simulink model "testing_C_functions_doubles3"  (R2020b)
settings: Solver=VariableStepAuto  StartTime=0.0  StopTime=2  FixedStep=Ts
undefined symbols (not defined in the file or in its folder): A_frq_step, A_phase_step, DiscIntNeverNeededParam, f_rad, k_phi, ki, kp, N, t_frq_step, t_phase_step, Ts, V_g, var_noise
libraries: simulink x9, bach_library x3, dspsrcs4 x2
settings Model: Creator=Kasper Laustsen  LastModifiedBy=Kasper Laustsen
settings SFSimCC: SimCustomHeaderCode=|
  | #include "PLL_doubled.h"
  | #include "MAF_doubled.h"
settings SFSimCC: SimUserSources=|
  | PLL_doubled.c
  | MAF_doubled.c

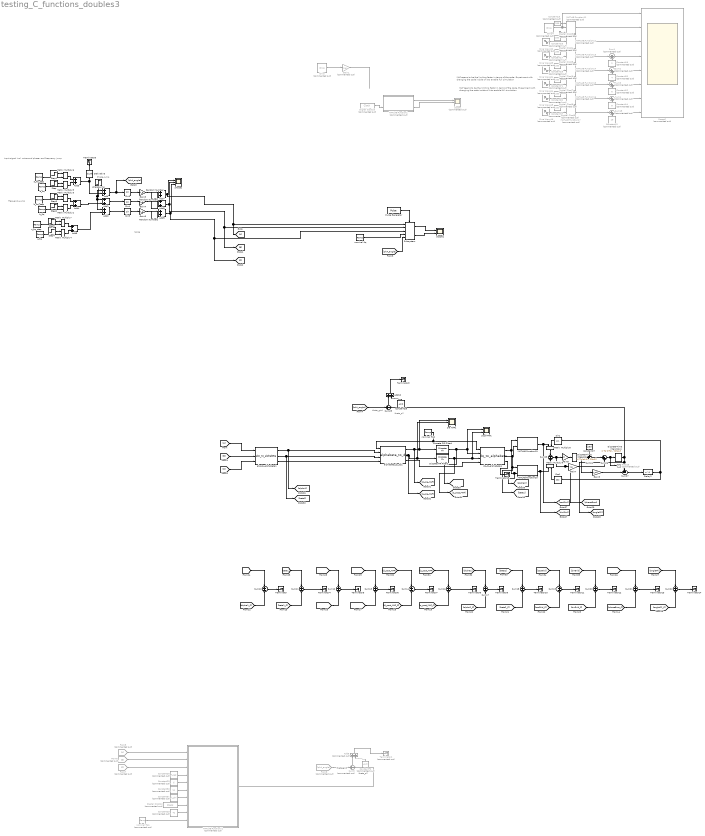
== system testing_C_functions_doubles3 ==
  note: MAF seems to be the limiting factor in terms of the code.
      | Experiment with changing the code inside of it to enable full simulation
  note: Noise
  note: Phase-jump
  note: Input signal incl. noise and phase- and frequency jump
  note: Frequency-jump
  note: MAF seems to be the limiting factor in terms of the code.
      | Experiment with changing the code inside of it to enable full simulation
  note: theta_pll
  note: theta_grid
  note: theta_pll
  note: theta_grid
  Add{,1..5,7..10} (10 alike) : Sum
  Add6 : Sum  Commented=on
  Chirp : dspsrcs4/Chirp  Commented=on  sweep=Linear  mode=Unidirectional  f0=0  f1=150  t1=3  Tsweep=3  phase=0  Ts=Ts  spf=1  datatype=Double  OutputFrames=off
  Chirp4 : dspsrcs4/Chirp  Commented=on  sweep=Linear  mode=Bidirectional  f0=0  f1=100  t1=2  Tsweep=2  phase=0  Ts=Ts  spf=1  datatype=Single  OutputFrames=off
  Constant12 : Constant  Commented=on  Value=6
  Constant13 : Constant  Commented=on  Value=10
  Constant14 : Constant  Commented=on  Value=8
  Constant{15..18,21..23} (7 alike) : Constant  Commented=on  Value=200
  Constant19 : Constant  Commented=on  Value=2
  Constant20 : Constant  Commented=on  Value=4
  Constant25 : Constant  Commented=on  Value=Ts
  Constant26 : Constant  Commented=on  Value=f_rad
  Constant27 : Constant  Value=f_rad
  Constant28 : Constant  Value=-pi/2
  Constant29 : Constant  Commented=on  Value=ki
  Constant30 : Constant  Commented=on  Value=kp
  Constant31 : Constant  Commented=on  Value=k_phi
  Constant32 : Constant  Commented=on  Value=-pi/2
  Cos1 : Trigonometry  Operator=cos
  Delay2 : Delay  DelayLength=1
  Derivative : Derivative
  Digital Clock{3..10,12} (9 alike) : DigitalClock  Commented=on  SampleTime=Ts
  Discrete FIR Filter2 : DiscreteFir  Coefficients=[ones(1,round(N)).*1/N]  SampleTime=Ts
  Discrete FIR Filter4 : DiscreteFir  Coefficients=[ones(1,round(N)).*1/N]  SampleTime=Ts
  Discrete-Time Integrator3 : DiscreteIntegrator  IntegratorMethod=Integration: Trapezoidal  SampleTime=-1  ICPrevOutput=DiscIntNeverNeededParam  ICPrevScaledInput=DiscIntNeverNeededParam
  Discrete-Time Integrator4 : DiscreteIntegrator  IntegratorMethod=Integration: Trapezoidal  SampleTime=-1  ICPrevOutput=DiscIntNeverNeededParam  ICPrevScaledInput=DiscIntNeverNeededParam
  From5 : From  Commented=on
  From6 : From  Commented=on  GotoTag=B
  From7 : From  Commented=on  GotoTag=C
  From8 : From  Commented=on  GotoTag=phA_angle
  Gain1 : Gain  Commented=on  Gain=V_g
  Gain3 : Gain  Gain=V_g
  Gain4 : Gain  Gain=V_g
  Gain5 : Gain  Gain=V_g
  Gain7 : Gain  Gain=kp
  Gain8 : Gain  Gain=ki
  Gain9 : Gain  Gain=k_phi
  Goto25 : Goto  Commented=on
  MATLAB Function1 : MATLAB Function  Commented=on  TreatAsAtomicUnit=on
  MATLAB Function11 : MATLAB Function  Commented=on  TreatAsAtomicUnit=on
  MATLAB Function12 : MATLAB Function  Commented=on  TreatAsAtomicUnit=on
  MATLAB Function13 : MATLAB Function  Commented=on  TreatAsAtomicUnit=on
  MATLAB Function14 : MATLAB Function  Commented=on  TreatAsAtomicUnit=on
  MATLAB Function15 : MATLAB Function  Commented=on  TreatAsAtomicUnit=on
  MATLAB Function16 : MATLAB Function  Commented=on  TreatAsAtomicUnit=on
  MATLAB Function17 : MATLAB Function  Commented=on  TreatAsAtomicUnit=on
  MATLAB Function19 : MATLAB Function  TreatAsAtomicUnit=on
  MATLAB Function20 : MATLAB Function  TreatAsAtomicUnit=on
  MATLAB Function21 : MATLAB Function  Commented=on  TreatAsAtomicUnit=on
  Matrix Multiply{2..9} (8 alike) : Product
  Pulse Generator : DiscretePulseGenerator  PulseType=Time based  Period=Ts  PulseWidth=50
  Random Number : RandomNumber  Variance=var_noise  SampleTime=Ts
  Random Number1 : RandomNumber  Variance=var_noise  Seed=1  SampleTime=Ts
  Random Number2 : RandomNumber  Variance=var_noise  Seed=2  SampleTime=Ts
  Scope : Scope  Commented=on  NumInputPorts=3
  Scope1 : Scope  NumInputPorts=2
  Scope2 : Scope  Commented=on  NumInputPorts=8
  Sin{1,3..5} (4 alike) : Trigonometry
  Sine Wave14 : Sin  Commented=on  Frequency=f_rad*2.6  Phase=pi/2  SampleTime=Ts
  Sine Wave15 : Sin  Commented=on  Frequency=f_rad*2.8  Phase=pi/2  SampleTime=Ts
  Sine Wave16 : Sin  Commented=on  Frequency=f_rad*3  Phase=pi/2  SampleTime=Ts
  Sine Wave22 : Sin  Commented=on  Frequency=f_rad*2  Phase=pi/2  SampleTime=Ts
  Sine Wave23 : Sin  Commented=on  Frequency=f_rad*2.2  Phase=pi/2  SampleTime=Ts
  Sine Wave24 : Sin  Commented=on  Frequency=f_rad*2.4  Phase=pi/2  SampleTime=Ts
  Step : Step  Time=t_frq_step  Before=1  After=0  SampleTime=0
  Step1 : Step  Time=t_frq_step  SampleTime=0
  Step2 : Step  Time=t_frq_step  Before=1  After=0  SampleTime=0
  Step3 : Step  Time=t_frq_step  SampleTime=0
  Step4 : Step  Time=t_frq_step  Before=1  After=0  SampleTime=0
  Step5 : Step  Time=t_frq_step  SampleTime=0
  Subsystem : Subsystem
  Sum{1..4,15} (5 alike) : Sum  Commented=on  Inputs=|++
  Sum{10..14,16..22,25} (13 alike) : Sum  Inputs=+|-
  Sum23 : Sum  Inputs=-|+
  Sum24 : Sum  Inputs=++|
  Sum26 : Sum  Inputs=|++
  Sum27 : Sum  Inputs=+-|
  Sum5 : Sum  Commented=on  Inputs=+|-
  Terminator{,2..15} (15 alike) : Terminator
  Terminator1 : Terminator  Commented=on
  a_frq : simulink/Sources/Ramp  slope=f_rad  start=0  InitialOutput=0
  a_frq_step : simulink/Sources/Ramp  slope=f_rad*A_frq_step  start=t_frq_step  InitialOutput=t_frq_step*f_rad
  abc_to_alphabeta1 : bach_library/abc_to_alphabeta  SystemSampleTime=-1  VariantActivationTime=update diagram  Latency=0  AutoFrameSizeCalculation=off
  alphabeta_to_dq1 : bach_library/alphabeta_to_dq  SystemSampleTime=-1  VariantActivationTime=update diagram  Latency=0  AutoFrameSizeCalculation=off
  b_frq : simulink/Sources/Ramp  slope=f_rad  start=0  InitialOutput=-pi*2/3
  b_frq_step : simulink/Sources/Ramp  slope=f_rad*A_frq_step  start=t_frq_step  InitialOutput=t_frq_step*f_rad-pi*2/3
  c_frq : simulink/Sources/Ramp  slope=f_rad  start=0  InitialOutput=pi*2/3
  c_frq_step : simulink/Sources/Ramp  slope=f_rad*A_frq_step  start=t_frq_step  InitialOutput=t_frq_step*f_rad+pi*2/3
  dq_to_alphabeta1 : bach_library/dq_to_alphabeta  SystemSampleTime=-1  VariantActivationTime=update diagram  Latency=0  AutoFrameSizeCalculation=off
  nominal frq : simulink/Sources/Ramp  slope=f_rad  start=0  InitialOutput=0
  nominal frq1 : simulink/Sources/Ramp  Commented=on  slope=f_rad  start=0  InitialOutput=0
  nominal frq2 : simulink/Sources/Ramp  slope=f_rad  start=0  InitialOutput=0
  phase-jump : Step  Time=t_phase_step  After=A_phase_step  SampleTime=0
  phases : Scope  NumInputPorts=3
  post MAF1 : Scope  NumInputPorts=2
  pre MAF1 : Scope  NumInputPorts=3
  wires:
  Matrix Multiply4/1 -> Add5/2
  Matrix Multiply6/1 -> Add3/1
  Step2/1 -> Matrix Multiply2/1
  Matrix Multiply7/1 -> Add5/1
  Step4/1 -> Matrix Multiply4/1
  a_frq_step/1 -> Matrix Multiply6/2
  a_frq/1 -> Matrix Multiply5/2
  Step/1 -> Matrix Multiply5/1
  Sin5/1 -> Gain5/1  "theta_g"
  Gain5/1 -> Add9/1  "pc"
  Step5/1 -> Matrix Multiply7/1
  Matrix Multiply2/1 -> Add4/2
  Add5/1 -> Add2/2  "c_phase"
  c_frq_step/1 -> Matrix Multiply7/2
  b_frq/1 -> Matrix Multiply2/2
  Gain4/1 -> Add8/1  "pb"
  phase-jump/1 -> Add/1, Add2/1, Add1/1
  Add4/1 -> Add1/2  "b_phase"
  Add3/1 -> Add/2, Derivative/1  "a_phase"
  Random Number2/1 -> Add9/2
  b_frq_step/1 -> Matrix Multiply3/2
  Gain3/1 -> Add7/1  "pa"
  Sin4/1 -> Gain4/1  "theta_g"
  Add1/1 -> Sin4/1
  Random Number/1 -> Add7/2
  c_frq/1 -> Matrix Multiply4/2
  Add2/1 -> Sin5/1
  Random Number1/1 -> Add8/2
  Sin3/1 -> Gain3/1  "theta_g"
  Matrix Multiply5/1 -> Add3/2
  Step3/1 -> Matrix Multiply3/1
  Matrix Multiply3/1 -> Add4/1
  Step1/1 -> Matrix Multiply6/1
  Derivative/1 -> Terminator3/1  "omega_g"
  Sum15/1 -> Scope2/8  "sin 150 Hz MAFed"
  Constant20/1 -> Sum2/2
  MATLAB Function12/1(y) -> Scope2/3  "sin 100 Hz MAFed"
  Constant19/1 -> Sum1/2
  MATLAB Function15/1(y) -> Sum3/1
  MATLAB Function14/1(y) -> Sum2/1
  Sine Wave14/1 -> MATLAB Function15/2(sample)
  Constant13/1 -> Sum15/2
  MATLAB Function17/1(y) -> Sum15/1
  MATLAB Function11/1(y) -> Scope2/2  "chirp MAFed"
  Sum2/1 -> Scope2/5  "sin 120 Hz MAFed"
  Sum3/1 -> Scope2/6  "sin 130 Hz MAFed"
  Chirp4/1 -> MATLAB Function11/2(sample), Scope2/1  "pa"
  Sine Wave22/1 -> MATLAB Function12/2(sample)
  Sine Wave15/1 -> MATLAB Function16/2(sample)
  MATLAB Function16/1(y) -> Sum4/1
  Sine Wave23/1 -> MATLAB Function13/2(sample)
  Constant14/1 -> Sum4/2
  Sum1/1 -> Scope2/4  "sin 110 Hz MAFed"
  MATLAB Function13/1(y) -> Sum1/1
  Sine Wave16/1 -> MATLAB Function17/2(sample)  "theta_g"
  Constant12/1 -> Sum3/2
  Sine Wave24/1 -> MATLAB Function14/2(sample)
  Sum4/1 -> Scope2/7  "sin 140 Hz MAFed"
  Constant15/1 -> MATLAB Function11/1(len)
  Digital Clock3/1 -> MATLAB Function11/3(t)
  Digital Clock4/1 -> MATLAB Function12/3(t)
  Constant16/1 -> MATLAB Function12/1(len)
  Digital Clock5/1 -> MATLAB Function13/3(t)
  Constant17/1 -> MATLAB Function13/1(len)
  Digital Clock6/1 -> MATLAB Function14/3(t)
  Constant18/1 -> MATLAB Function14/1(len)
  Digital Clock7/1 -> MATLAB Function15/3(t)
  Constant21/1 -> MATLAB Function15/1(len)
  Digital Clock8/1 -> MATLAB Function16/3(t)
  Constant22/1 -> MATLAB Function16/1(len)
  Digital Clock9/1 -> MATLAB Function17/3(t)
  Constant23/1 -> MATLAB Function17/1(len)
  Chirp/1 -> Gain1/1  "chirp"
  Gain1/1 -> ?  "pa"
  [alpha1] -> Sum10/1
  [alpha1_C] -> Sum10/2
  [beta1] -> Sum11/1
  [beta1_C] -> Sum11/2
  [d_pre_MAF] -> Sum12/1
  [d_pre_MAF_C] -> Sum12/2
  [q_pre_MAF_C] -> Sum13/2
  [q_pre_MAF] -> Sum13/1
  [d_post_MAF] -> Sum14/1
  [d_post_MAF_C] -> Sum14/2
  [q_post_MAF] -> Sum16/1
  [q_post_MAF_C] -> Sum16/2
  [alpha2] -> Sum17/1
  [alpha2_C] -> Sum17/2
  [beta2] -> Sum18/1
  [beta2_C] -> Sum18/2
  [cosGrid] -> Sum19/1
  [cosGrid_C] -> Sum19/2
  [sinGrid] -> Sum20/1
  [sinGrid_C] -> Sum20/2
  [phaseError] -> Sum21/1
  [phaseError_C] -> Sum21/2
  [anglePll] -> Sum22/1
  [anglePll_C] -> Sum22/2
  Sum10/1 -> Terminator/1  "diff_alpha1"
  Sum11/1 -> Terminator4/1  "diff_beta1"
  Sum12/1 -> Terminator5/1  "diff_d_pre_MAF"
  Sum13/1 -> Terminator6/1  "diff_q_pre_MAF"
  Sum14/1 -> Terminator7/1  "diff_d_post_MAF"
  Sum16/1 -> Terminator8/1  "diff_q_post_MAF"
  Sum17/1 -> Terminator9/1  "diff_alpha2"
  Sum18/1 -> Terminator10/1  "diff_beta2"
  Sum19/1 -> Terminator11/1  "diff_cosGrid"
  Sum20/1 -> Terminator12/1  "diff_sinGrid"
  Sum21/1 -> Terminator13/1  "diff_phaseError"
  Sum22/1 -> Terminator14/1  "diff_anglePll"
  Sum27/1 -> Delay2/1  "theta_comp"
  Sum25/1 -> Add10/1  "theta_err_sim"
  alphabeta_to_dq1/3 -> dq_to_alphabeta1/4
  Gain7/1 -> Sum26/2
  Gain8/1 -> Discrete-Time Integrator3/1
  Constant27/1 -> Sum24/1
  dq_to_alphabeta1/3 -> Terminator15/1
  Cos1/1 -> Matrix Multiply9/2  "cos_pll"
  MATLAB Function20/1(sin_grid) -> [sinGrid], Matrix Multiply9/1  "sin_grid"
  Gain9/1 -> Sum27/2  "k_phi"
  Add/1 -> [phA_angle], Sin3/1  "pha_angle"
  abc_to_alphabeta1/3 -> alphabeta_to_dq1/4
  abc_to_alphabeta1/1 -> alphabeta_to_dq1/2, [alpha1]  "alpha1"
  Discrete FIR Filter4/1 -> [d_post_MAF], post MAF1/1, dq_to_alphabeta1/2  "d_post_MAF"
  abc_to_alphabeta1/2 -> alphabeta_to_dq1/3, [beta1]  "beta1"
  dq_to_alphabeta1/2 -> [beta2], MATLAB Function20/1(beta), MATLAB Function19/2(beta)  "beta2"
  nominal frq2/1 -> dq_to_alphabeta1/1, alphabeta_to_dq1/1
  Add8/1 -> phases/2, [B], Subsystem/2(pb)  "pb"
  Sin1/1 -> Matrix Multiply8/2  "sin_pll"
  Discrete-Time Integrator4/1 -> Sum27/1, [anglePll], Sum25/2  "theta"
  Sum24/1 -> Sum26/1
  alphabeta_to_dq1/1 -> [d_pre_MAF], pre MAF1/1, Discrete FIR Filter4/1  "d_pre_MAF"
  Sum26/1 -> Discrete-Time Integrator4/1, Goto25/1  "omega"
  Discrete FIR Filter2/1 -> [q_post_MAF], post MAF1/2, dq_to_alphabeta1/3  "q_post_MAF"
  Add10/1 -> Terminator2/1  "theta_err_sim_offset_delay"
  Matrix Multiply9/1 -> Sum23/2  "sin_grid_cos_pll"
  alphabeta_to_dq1/2 -> [q_pre_MAF], Discrete FIR Filter2/1, pre MAF1/2  "q_pre_MAF"
  dq_to_alphabeta1/1 -> MATLAB Function19/1(alpha), [alpha2], MATLAB Function20/2(alpha)  "alpha2"
  Add9/1 -> Subsystem/3(pc), [C], phases/3  "pc"
  Matrix Multiply8/1 -> Sum23/1  "cos_grid_sin_pll"
  Constant28/1 -> Add10/2
  Discrete-Time Integrator3/1 -> Sum24/2, Gain9/1
  Add7/1 -> [A], Subsystem/1(pa), phases/1  "pa"
  MATLAB Function19/1(cos_grid) -> [cosGrid], Matrix Multiply8/1  "cos_grid"
  Sum23/1 -> Gain8/1, [phaseError], Gain7/1  "phaseError"
  Delay2/1 -> Sin1/1, Cos1/1
  [phA_angle] -> Sum25/1
  [C] -> abc_to_alphabeta1/3
  [B] -> abc_to_alphabeta1/2
  [A] -> abc_to_alphabeta1/1
  Digital Clock10/1 -> MATLAB Function1/3(t)
  MATLAB Function1/1(y1) -> Scope/1  "d_post_maf_C"
  MATLAB Function1/2(y2) -> Scope/2  "q_post_maf_C"
  Constant25/1 -> MATLAB Function21/9(Ts)
  Constant30/1 -> MATLAB Function21/6(kp)
  Constant31/1 -> MATLAB Function21/7(kPhi)
  Constant29/1 -> MATLAB Function21/5(ki)
  Constant26/1 -> MATLAB Function21/4(feedForward)
  Digital Clock12/1 -> MATLAB Function21/8(t)
  From7/1 -> MATLAB Function21/3(c)
  From6/1 -> MATLAB Function21/2(b)
  From5/1 -> MATLAB Function21/1(a)
  nominal frq1/1 -> MATLAB Function21/10(angle)
  From8/1 -> Sum5/1
  Add6/1 -> Terminator1/1  "Angle Error C sammensat"
  Sum5/1 -> Add6/1  "theta_err_sim"
  MATLAB Function21/1(anglePll) -> Sum5/2  "theta"
  Constant32/1 -> Add6/2
  Pulse Generator/1 -> Subsystem/Trigger
  nominal frq/1 -> Subsystem/4("angle ")
  [phA_angle] -> Subsystem/5(True phase angle A)  "True angle"
  Subsystem/1(Out1) -> Scope1/1  "Angle Error C"
  Subsystem/2(anglePll) -> Scope1/2  "Angle Pll triggered"

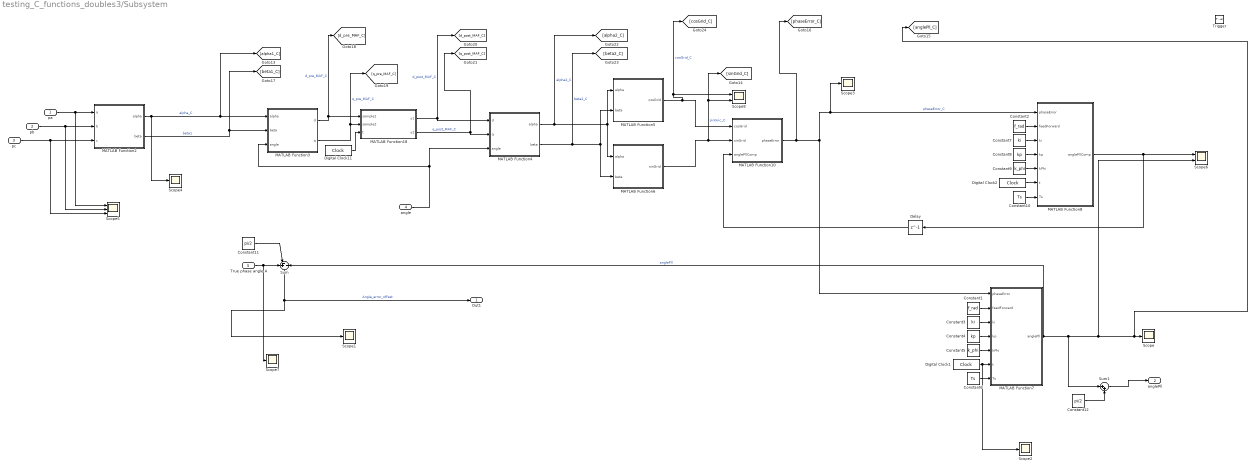
== system testing_C_functions_doubles3/Subsystem ==
  pa : Inport
  pb : Inport  Port=2
  pc : Inport  Port=3
  "angle " : Inport  Port=4
  True phase angle A : Inport  Port=5
  Trigger : TriggerPort  VariantControl=Variant  PortDimensions=1
  Constant1 : Constant  Value=f_rad
  Constant10 : Constant  Value=Ts
  Constant11 : Constant  Value=pi/2
  Constant12 : Constant  Value=pi/2
  Constant2 : Constant  Value=f_rad
  Constant3 : Constant  Value=ki
  Constant4 : Constant  Value=kp
  Constant5 : Constant  Value=k_phi
  Constant6 : Constant  Value=Ts
  Constant7 : Constant  Value=ki
  Constant8 : Constant  Value=kp
  Constant9 : Constant  Value=k_phi
  Delay : Delay  DelayLength=1
  Digital Clock1 : DigitalClock  SampleTime=-1
  Digital Clock11 : DigitalClock  SampleTime=-1
  Digital Clock2 : DigitalClock  SampleTime=-1
  MATLAB Function10 : MATLAB Function  TreatAsAtomicUnit=on
  MATLAB Function18 : MATLAB Function  TreatAsAtomicUnit=on
  MATLAB Function2 : MATLAB Function  TreatAsAtomicUnit=on
  MATLAB Function3 : MATLAB Function  TreatAsAtomicUnit=on
  MATLAB Function4 : MATLAB Function  TreatAsAtomicUnit=on
  MATLAB Function5 : MATLAB Function  TreatAsAtomicUnit=on
  MATLAB Function6 : MATLAB Function  TreatAsAtomicUnit=on
  MATLAB Function7 : MATLAB Function  TreatAsAtomicUnit=on
  MATLAB Function8 : MATLAB Function  TreatAsAtomicUnit=on
  Scope{,1..4,7} (6 alike) : Scope
  Scope5 : Scope  NumInputPorts=3
  Scope6 : Scope  NumInputPorts=2
  Scope8 : Scope  NumInputPorts=2
  Sum : Sum  Inputs=+-|-
  Sum1 : Sum  Inputs=|++
  Out1 : Outport
  anglePll : Outport  Port=2
  wires:
  MATLAB Function5/1(cosGrid) -> [cosGrid_C], Scope8/1, MATLAB Function10/1(cosGrid)  "cosGrid_C"
  MATLAB Function2/1(alpha) -> [alpha1_C], MATLAB Function3/1(alpha), Scope4/1  "alpha_C"
  MATLAB Function7/1(anglePll) -> Sum/3, Sum1/1, Scope6/2, Scope/1, [anglePll_C]  "anglePll"
  Constant10/1 -> MATLAB Function8/7(Ts)
  Delay/1 -> MATLAB Function10/3(anglePllComp)
  MATLAB Function6/1(sinGrid) -> MATLAB Function10/2(sinGrid), Scope8/2, [sinGrid_C]  "sinGric_C"
  MATLAB Function4/1(alpha) -> [alpha2_C], MATLAB Function5/1(alpha), MATLAB Function6/1(alpha)  "alpha2_C"
  True phase angle A/1 -> Scope7/1, Sum/1
  Constant7/1 -> MATLAB Function8/3(ki)
  Digital Clock1/1 -> Scope2/1, MATLAB Function7/6(t)
  MATLAB Function18/2(y2) -> [q_post_MAF_C], MATLAB Function4/2(q)  "q_post_MAF_C"
  MATLAB Function4/2(beta) -> [beta2_C], MATLAB Function5/2(beta), MATLAB Function6/2(beta)  "beta2_C"
  Digital Clock2/1 -> MATLAB Function8/6(t)
  Digital Clock11/1 -> MATLAB Function18/3(t)
  MATLAB Function2/2(beta) -> MATLAB Function3/2(beta), [beta1_C]  "beta1"
  Constant5/1 -> MATLAB Function7/5(kPhi)
  Constant3/1 -> MATLAB Function7/3(ki)
  Constant8/1 -> MATLAB Function8/4(kp)
  Constant1/1 -> MATLAB Function7/2(feedForward)
  Constant2/1 -> MATLAB Function8/2(feedForward)
  pa/1 -> Scope5/1, MATLAB Function2/1(a)
  MATLAB Function10/1(phaseError) -> [phaseError_C], MATLAB Function7/1(phaseError), Scope3/1, MATLAB Function8/1(phaseError)  "phaseError_C"
  MATLAB Function18/1(y1) -> [d_post_MAF_C], MATLAB Function4/1(d)  "d_post_MAF_C"
  MATLAB Function3/2(q) -> MATLAB Function18/2(sample2), [q_pre_MAF_C]  "q_pre_MAF_C"
  Constant9/1 -> MATLAB Function8/5(kPhi)
  Constant4/1 -> MATLAB Function7/4(kp)
  MATLAB Function3/1(d) -> MATLAB Function18/1(sample1), [d_pre_MAF_C]  "d_pre_MAF_C"
  "angle "/1 -> MATLAB Function3/3(angle), MATLAB Function4/3(angle)
  Constant11/1 -> Sum/2
  Constant6/1 -> MATLAB Function7/7(Ts)
  MATLAB Function8/1(anglePllComp) -> Delay/1, Scope6/1
  Sum/1 -> Out1/1, Scope1/1  "Angle_error_offset"
  pc/1 -> Scope5/3, MATLAB Function2/3(c)
  pb/1 -> Scope5/2, MATLAB Function2/2(b)
  Constant12/1 -> Sum1/2
  Sum1/1 -> anglePll/1

== matlab function testing_C_functions_doubles3/Subsystem/MATLAB Function10 ==
  data: cosGrid input; phaseError output; sinGrid input; anglePllComp input
function phaseError  = calling_phase_detector(cosGrid, sinGrid, anglePllComp)
% coder.updateBuildInfo('addSourceFiles','abc_to_alphabeta.c');
% coder.cinclude('abc_to_alphabeta.h');
coder.updateBuildInfo('addSourceFiles','PLL_doubled.c');
coder.cinclude('PLL_doubled.h');

phaseError = 0.0;

phaseError = coder.ceval('phase_detector', cosGrid, sinGrid, anglePllComp);

== matlab function testing_C_functions_doubles3/MATLAB Function11 ==
  data: len input; sample input; y output; t input
function y = calling_moving_avg(len, sample, t)
% coder.updateBuildInfo('addSourceFiles','moving_avg.c');
% coder.cinclude('moving_avg.h');

coder.updateBuildInfo('addSourceFiles','MAF.c');
coder.cinclude('MAF.h');

y = 0.0;
% y = coder.ceval('moving_avg',u,t);
y = coder.ceval('maf',len, sample, t);

== matlab function testing_C_functions_doubles3/MATLAB Function12 ==
  data: len input; sample input; y output; t input
function y = calling_moving_avg(len, sample, t)
% coder.updateBuildInfo('addSourceFiles','moving_avg.c');
% coder.cinclude('moving_avg.h');

coder.updateBuildInfo('addSourceFiles','MAF.c');
coder.cinclude('MAF.h');

y = 0.0;
% y = coder.ceval('moving_avg',u,t);
y = coder.ceval('maf',len, sample, t);

== matlab function testing_C_functions_doubles3/MATLAB Function13 ==
  data: len input; sample input; y output; t input
function y = calling_moving_avg(len, sample, t)
% coder.updateBuildInfo('addSourceFiles','moving_avg.c');
% coder.cinclude('moving_avg.h');

coder.updateBuildInfo('addSourceFiles','MAF.c');
coder.cinclude('MAF.h');

y = 0.0;
% y = coder.ceval('moving_avg',u,t);
y = coder.ceval('maf',len, sample, t);

== matlab function testing_C_functions_doubles3/MATLAB Function14 ==
  data: len input; sample input; y output; t input
function y = calling_moving_avg(len, sample, t)
% coder.updateBuildInfo('addSourceFiles','moving_avg.c');
% coder.cinclude('moving_avg.h');

coder.updateBuildInfo('addSourceFiles','MAF.c');
coder.cinclude('MAF.h');

y = 0.0;
% y = coder.ceval('moving_avg',u,t);
y = coder.ceval('maf',len, sample, t);

== matlab function testing_C_functions_doubles3/MATLAB Function15 ==
  data: len input; sample input; y output; t input
function y = calling_moving_avg(len, sample, t)
% coder.updateBuildInfo('addSourceFiles','moving_avg.c');
% coder.cinclude('moving_avg.h');

coder.updateBuildInfo('addSourceFiles','MAF.c');
coder.cinclude('MAF.h');

y = 0.0;
% y = coder.ceval('moving_avg',u,t);
y = coder.ceval('maf',len, sample, t);

== matlab function testing_C_functions_doubles3/MATLAB Function16 ==
  data: len input; sample input; y output; t input
function y = calling_moving_avg(len, sample, t)
% coder.updateBuildInfo('addSourceFiles','moving_avg.c');
% coder.cinclude('moving_avg.h');

coder.updateBuildInfo('addSourceFiles','MAF.c');
coder.cinclude('MAF.h');

y = 0.0;
% y = coder.ceval('moving_avg',u,t);
y = coder.ceval('maf',len, sample, t);

== matlab function testing_C_functions_doubles3/MATLAB Function17 ==
  data: len input; sample input; y output; t input
function y = calling_moving_avg(len, sample, t)
% coder.updateBuildInfo('addSourceFiles','moving_avg.c');
% coder.cinclude('moving_avg.h');

coder.updateBuildInfo('addSourceFiles','MAF.c');
coder.cinclude('MAF.h');

y = 0.0;
% y = coder.ceval('moving_avg',u,t);
y = coder.ceval('maf',len, sample, t);

== matlab function testing_C_functions_doubles3/Subsystem/MATLAB Function18 ==
  data: sample1 input; sample2 input; y1 output; t input; y2 output
function [y1, y2] = calling_moving_avg(sample1, sample2, t)
% coder.updateBuildInfo('addSourceFiles','moving_avg.c');
% coder.cinclude('moving_avg.h');

coder.updateBuildInfo('addSourceFiles','MAF_doubled.c');
coder.cinclude('MAF_doubled.h');

y1 = 0.0;
y2 = 0.0;
% y = coder.ceval('moving_avg',u,t);
% y1 = coder.ceval('maf1',len, sample1, t);
% y2 = coder.ceval('maf2',len, sample2, t);
y1 = coder.ceval('maf1', sample1, t); %explicit def of length removed
y2 = coder.ceval('maf2', sample2, t); %explicit def of length removed

== matlab function testing_C_functions_doubles3/MATLAB Function1 ==
  data: sample1 input; sample2 input; y1 output; t input; y2 output
function [y1, y2] = calling_moving_avg(sample1, sample2, t)
% coder.updateBuildInfo('addSourceFiles','moving_avg.c');
% coder.cinclude('moving_avg.h');

coder.updateBuildInfo('addSourceFiles','MAF_doubled.c');
coder.cinclude('MAF_doubled.h');

y1 = 0.0;
y2 = 0.0;
% y = coder.ceval('moving_avg',u,t);
% y1 = coder.ceval('maf1',len, sample1, t);
% y2 = coder.ceval('maf2',len, sample2, t);
y1 = coder.ceval('maf1', sample1, t); %explicit def of length removed
y2 = coder.ceval('maf2', sample2, t); %explicit def of length removed

== matlab function testing_C_functions_doubles3/MATLAB Function21 ==
  data: a input; b input; c input; anglePll output; feedForward input; ki input; kp input; kPhi input; t input; Ts input; angle input
function anglePll  = calling_pll(a, b, c, feedForward, ki, kp, kPhi, t, Ts, angle)
% coder.updateBuildInfo('addSourceFiles','abc_to_alphabeta.c');
% coder.cinclude('abc_to_alphabeta.h');
coder.updateBuildInfo('addSourceFiles','PLL.c');
coder.cinclude('PLL.h');

anglePll = 0.0;

anglePll = coder.ceval('pll', a, b, c, feedForward, ki, kp, kPhi, t, Ts, angle);

== matlab function testing_C_functions_doubles3/MATLAB Function19 ==
  data: alpha input; cos_grid output; beta input
function cos_grid = cos_grid(alpha, beta)

cos_grid = alpha/sqrt(alpha^2+beta^2);

== matlab function testing_C_functions_doubles3/MATLAB Function20 ==
  data: beta input; alpha input; sin_grid output
function sin_grid = sin_grid(beta, alpha)

sin_grid = beta/sqrt(alpha^2+beta^2);

== matlab function testing_C_functions_doubles3/Subsystem/MATLAB Function2 ==
  data: a input; alpha output; b input; c input; beta output
function [alpha,beta] = calling_abc_to_alphabeta(a,b,c)
% coder.updateBuildInfo('addSourceFiles','abc_to_alphabeta.c');
% coder.cinclude('abc_to_alphabeta.h');
coder.updateBuildInfo('addSourceFiles','PLL_doubled.c');
coder.cinclude('PLL_doubled.h');


alpha = 0.0;
beta = 0.0;

alpha = coder.ceval('abc_to_alpha',a,b,c);
beta = coder.ceval('abc_to_beta',a,b,c);

== matlab function testing_C_functions_doubles3/Subsystem/MATLAB Function3 ==
  data: alpha input; d output; beta input; angle input; q output
function [d, q] = calling_alphabeta_to_dq(alpha, beta, angle)
% coder.updateBuildInfo('addSourceFiles','abc_to_alphabeta.c');
% coder.cinclude('abc_to_alphabeta.h');
coder.updateBuildInfo('addSourceFiles','PLL_doubled.c');
coder.cinclude('PLL_doubled.h');


d = 0.0;
q = 0.0;

d = coder.ceval('alphabeta_to_d',alpha, beta, angle);
q = coder.ceval('alphabeta_to_q',alpha, beta, angle);

== matlab function testing_C_functions_doubles3/Subsystem/MATLAB Function4 ==
  data: d input; alpha output; q input; angle input; beta output
function [alpha, beta] = calling_dq_to_alphabeta(d, q, angle)
% coder.updateBuildInfo('addSourceFiles','abc_to_alphabeta.c');
% coder.cinclude('abc_to_alphabeta.h');
coder.updateBuildInfo('addSourceFiles','PLL_doubled.c');
coder.cinclude('PLL_doubled.h');


alpha = 0.0;
beta = 0.0;

alpha = coder.ceval('dq_to_alpha', d, q, angle);
beta = coder.ceval('dq_to_beta', d, q, angle);

== matlab function testing_C_functions_doubles3/Subsystem/MATLAB Function5 ==
  data: alpha input; cosGrid output; beta input
function cosGrid  = calling_cos_grid(alpha, beta)
% coder.updateBuildInfo('addSourceFiles','abc_to_alphabeta.c');
% coder.cinclude('abc_to_alphabeta.h');
coder.updateBuildInfo('addSourceFiles','PLL_doubled.c');
coder.cinclude('PLL_doubled.h');

cosGrid = 0.0;

cosGrid = coder.ceval('cos_grid', alpha, beta);

== matlab function testing_C_functions_doubles3/Subsystem/MATLAB Function6 ==
  data: alpha input; sinGrid output; beta input
function sinGrid  = calling_sin_grid(alpha, beta)
% coder.updateBuildInfo('addSourceFiles','abc_to_alphabeta.c');
% coder.cinclude('abc_to_alphabeta.h');
coder.updateBuildInfo('addSourceFiles','PLL_doubled.c');
coder.cinclude('PLL_doubled.h');

sinGrid = 0.0;

sinGrid = coder.ceval('sin_grid', alpha, beta);

== matlab function testing_C_functions_doubles3/Subsystem/MATLAB Function7 ==
  data: phaseError input; anglePll output; feedForward input; ki input; kp input; kPhi input; t input; Ts input
function anglePll  = calling_pi_regulator(phaseError, feedForward, ki, kp, kPhi, t, Ts)
% coder.updateBuildInfo('addSourceFiles','abc_to_alphabeta.c');
% coder.cinclude('abc_to_alphabeta.h');
coder.updateBuildInfo('addSourceFiles','PLL_doubled.c');
coder.cinclude('PLL_doubled.h');

anglePll = 0.0;

anglePll = coder.ceval('pi_regulator', phaseError, feedForward, ki, kp, kPhi, t, Ts);

== matlab function testing_C_functions_doubles3/Subsystem/MATLAB Function8 ==
  data: phaseError input; anglePllComp output; feedForward input; ki input; kp input; kPhi input; t input; Ts input
function anglePllComp  = calling_pi_regulator_comp(phaseError, feedForward, ki, kp, kPhi, t, Ts)
% coder.updateBuildInfo('addSourceFiles','abc_to_alphabeta.c');
% coder.cinclude('abc_to_alphabeta.h');
coder.updateBuildInfo('addSourceFiles','PLL_doubled.c');
coder.cinclude('PLL_doubled.h');

anglePllComp = 0.0;

anglePllComp = coder.ceval('pi_regulator_comp', phaseError, feedForward, ki, kp, kPhi, t, Ts);
